simulink model "Yaw_simulink_lqr"  (R2018b)
settings: Solver=VariableStepAuto  StartTime=0.0  StopTime=7  RelTol=1e-3
values from neighbouring files (symbols this model uses):
  beta = 63.4*pi/180    (= 1.10653874576)    [Spacecraft.m]
  int_resist = 50    [Spacecraft.m]
  Iw = max([Iw_roll Iw_pitch Iw_yaw])    [Spacecraft.m]    (also in maneuver.m = z2(end)*Is/(4*Omega_max*cos(beta)))
  Izz = 50000    [Spacecraft.m]
  yaw_accu = 0.05    [Spacecraft.m]
undefined symbols (not defined in the file or in its folder): Ap, Bp, Cp, Dp, Ky, N, phi_yaw
libraries: simulink x1
settings Model: Creator=Utilisateur  LastModifiedBy=Utilisateur

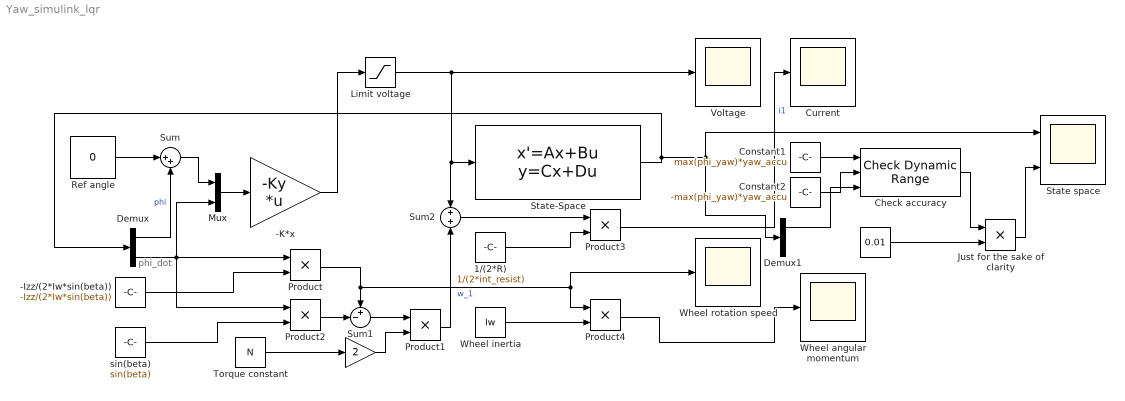
== system Yaw_simulink_lqr ==
  note: phi_dot
  " " : Constant  Value=0.01
  " " : Gain  Gain=2
  -Izz/(2*Iw*sin(beta)) : Constant  Value=-Izz/(2*Iw*sin(beta))
  "-K*x " : Gain  Gain=-Ky  Multiplication=Matrix(K*u) (u vector)
  1/(2*R) : Constant  Value=1/(2*int_resist)
  Check accuracy : simulink/Model Verification/Check  Dynamic Range  Description=min < u < max  enabled=on  stopWhenAssertionFail=off  export=on  icon=graphic
      settings: SourceProductName=Simulink  SourceProductBaseCode=SL
  Constant1 : Constant  Value=max(phi_yaw)*yaw_accu
  Constant2 : Constant  Value=-max(phi_yaw)*yaw_accu
  Current : Scope
  Demux : Demux  Outputs=2
  Demux1 : Demux  Outputs=2
  Just for the sake of clarity : Product
  Limit voltage : Saturate  UpperLimit=900  LowerLimit=-900
  Mux : Mux  Inputs=2
  Product{,1..4} (5 alike) : Product
  Ref angle : Constant  Value=0
  State space : Scope  NumInputPorts=2
  State-Space : StateSpace  A=Ap  B=Bp  C=Cp  D=Dp  InitialCondition=[max(phi_yaw);0]
  Sum : Sum  Inputs=|++
  Sum1 : Sum  Inputs=+-|
  Sum2 : Sum  Inputs=+|+
  Torque constant : Constant  Value=N
  Voltage : Scope
  Wheel angular momentum : Scope
  Wheel inertia : Constant  Value=Iw
  Wheel rotation speed : Scope
  sin(beta) : Constant  Value=sin(beta)
  wires:
  Sum/1 -> Mux/1
  Sum1/1 -> Product1/1
  -Izz/(2*Iw*sin(beta))/1 -> Product/2
  "-K*x "/1 -> Limit voltage/1
  Mux/1 -> "-K*x "/1
  Product3/1 -> Current/1  "i1"
  Product1/1 -> Sum2/2
  Product4/1 -> Wheel angular momentum/1
  Wheel inertia/1 -> Product4/2
  " "/1 -> Product1/2
  State-Space/1 -> Demux1/1, State space/1, Demux/1
  Torque constant/1 -> " "/1
  Ref angle/1 -> Sum/1
  1/(2*R)/1 -> Product3/2
  Demux/2 -> Product/1, Mux/2, Product2/1
  sin(beta)/1 -> Product2/2
  Sum2/1 -> Product3/1
  Demux/1 -> Sum/2  "phi"
  Limit voltage/1 -> Sum2/1, State-Space/1, Voltage/1
  Product2/1 -> Sum1/2
  Product/1 -> Product4/1, Wheel rotation speed/1, Sum1/1  "w_1"
  Constant1/1 -> Check accuracy/1
  Check accuracy/1 -> Just for the sake of clarity/1
  Demux1/1 -> Check accuracy/3
  Constant2/1 -> Check accuracy/2
  " "/1 -> Just for the sake of clarity/2
  Just for the sake of clarity/1 -> State space/2
